simulink model "untitled"  (R2017b)
settings: Solver=FixedStepDiscrete  StartTime=0.0  StopTime=10.0  FixedStep=0.1  RelTol=1e-3  EnableMultiTasking=on
libraries: frdmk64flib x4, xpcutilitieslib x1
settings Model: ExtModeTrigDuration=5  Creator=yuy61  LastModifiedBy=chengm15
settings SolverCC: AutoInsertRateTranBlk=on
settings DataIOCC: LimitDataPoints=on
settings OptimizationCC: PassReuseOutputArgsAs=Individual arguments  MaxStackSize=64
settings DebuggingCC: ParameterTunabilityLossMsg=error  AllowSymbolicDim=off  SFUnexpectedBacktrackingDiag=warning  SFNoUnconditionalDefaultTransitionDiag=warning  SFExecutionAtInitializationDiag=none
settings HardwareCC: ProdBitPerPointer=32  ProdBitPerSizeT=32  ProdBitPerPtrDiffT=32  ProdLargestAtomicInteger=Long  ProdLargestAtomicFloat=Double  ProdWordSize=32  ProdHWDeviceType=ARM Compatible->ARM Cortex
settings SFSimCC: MATLABDynamicMemAlloc=off
settings RTWCC: SystemTargetFile=ert.tlc  HardwareBoard=NXP FRDM-K64F  TemplateMakefile=ert_default_tmf  GenerateReport=on  Toolchain=GNU Tools for ARM Embedded Processors  IncludeHyperlinkInReport=on  LaunchReport=on  GenerateTraceInfo=on  GenerateTraceReport=on  GenerateTraceReportSl=on  GenerateTraceReportSf=on  GenerateTraceReportEml=on
settings CodeAppCC: ForceParamTrailComments=on  IgnoreCustomStorageClasses=off  OperatorAnnotations=on  SimulinkDataObjDesc=on  SFDataObjDesc=on  InsertBlockDesc=on
settings ConfigComp: CovMetricSettings=dw  CovHtmlReporting=on  CovSaveCumulativeToWorkspaceVar=on  CovSaveSingleToWorkspaceVar=on  CovShowResultsExplorer=off  CovExternalEMLEnable=off  CovSFcnEnable=off

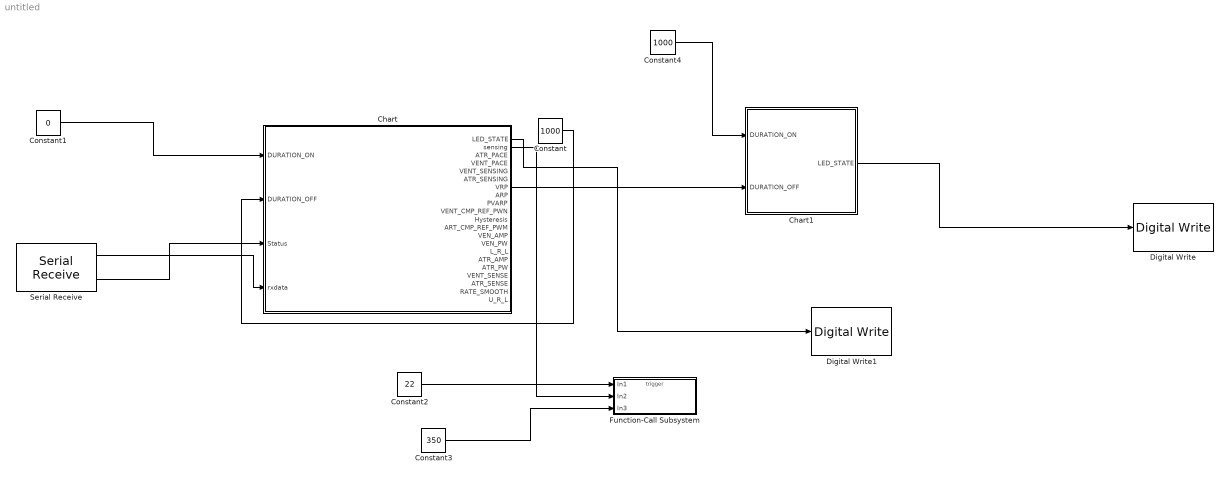
== system untitled ==
  Chart : Stateflow chart  TreatAsAtomicUnit=on
  Chart1 : Stateflow chart  TreatAsAtomicUnit=on
  Constant : Constant  Value=1000  OutDataTypeStr=int16
  Constant1 : Constant  Value=0  OutDataTypeStr=int16
  Constant2 : Constant  Value=22  OutDataTypeStr=uint8
  Constant3 : Constant  Value=350  VectorParams1D=off  OutDataTypeStr=uint16
  Constant4 : Constant  Value=1000  OutDataTypeStr=uint16
  Digital Write : frdmk64flib/Digital Write  Whichpin=RED_LED
      settings: SourceProductName=Simulink Coder Support Package for NXP FRDM-K64F Board
  Digital Write1 : frdmk64flib/Digital Write  Whichpin=GREEN_LED
      settings: SourceProductName=Simulink Coder Support Package for NXP FRDM-K64F Board
  Function-Call Subsystem : Subsystem  TreatAsAtomicUnit=on
  Serial Receive : frdmk64flib/Serial Receive  SCIModule=0  Baudrate=uint32(9600)  Parity=None  StopBits=1  HardwareFlowControl=None  ByteOrder=LittleEndian  DataType=uint8  DataLength=23  BlockingMode=off  OutputStatus=on  SampleTime=-1
      settings: SourceProductName=Simulink Coder Support Package for NXP FRDM-K64F Board
  wires:
  Constant/1 -> Chart/2(DURATION_OFF)
  Constant1/1 -> Chart/1(DURATION_ON)
  Serial Receive/2 -> Chart/3(Status)
  Serial Receive/1 -> Chart/4(rxdata)
  Chart/2(sensing) -> Function-Call Subsystem/2(In2)
  Constant2/1 -> Function-Call Subsystem/1(In1)
  Constant3/1 -> Function-Call Subsystem/3(In3)
  Chart1/1(LED_STATE) -> Digital Write/1
  Chart/7(VRP) -> Chart1/2(DURATION_OFF)
  Constant4/1 -> Chart1/1(DURATION_ON)
  Chart/1(LED_STATE) -> Digital Write1/1

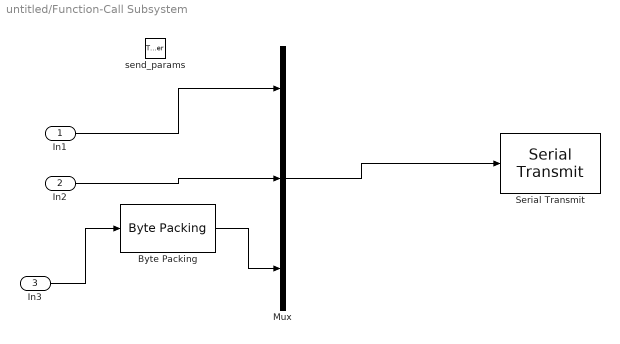
== system untitled/Function-Call Subsystem ==
  In1 : Inport  OutDataTypeStr=uint8
  In2 : Inport  Port=2  OutDataTypeStr=uint8
  In3 : Inport  Port=3  OutDataTypeStr=uint16
  send_params : TriggerPort  TriggerType=function-call  IsSimulinkFunction=on  FunctionName=send_params  VariantControl=Variant
  "Byte Packing " : xpcutilitieslib/Byte Packing   MaskPackedDataType=uint8  MaskUnpackedDataTypes={'uint16'}  MaskAlignment=1
  Mux : Mux  Inputs=3
  Serial Transmit : frdmk64flib/Serial Transmit  SCIModule=0  Baudrate=uint32(9600)  Parity=None  StopBits=1  HardwareFlowControl=None  ByteOrder=LittleEndian  BlockingMode=on  OutputStatus=off
      settings: SourceProductName=Simulink Coder Support Package for NXP FRDM-K64F Board
  wires:
  In1/1 -> Mux/1
  In2/1 -> Mux/2
  Mux/1 -> Serial Transmit/1
  In3/1 -> "Byte Packing "/1
  "Byte Packing "/1 -> Mux/3

== stateflow chart untitled/Chart1 ==
  state LED_ON
    entry:
    LED_STATE = true;
  state LED_OFF
    entry:
    LED_STATE = false;
  (default) -> LED_ON
  LED_ON -> LED_OFF : [DURATION_OFF == hex2dec('15E')]
  LED_OFF -> LED_ON : [after(DURATION_ON,msec)]
  data: DURATION_ON input uint16; DURATION_OFF input uint16; LED_STATE output boolean

== stateflow chart untitled/Chart ==
  settings: executeAtInitialization=1
  state LED_OFF
    entry:
    LED_STATE = false;
    ATR_PACE = rxdata(2)
    VENT_PACE = rxdata(3)
    ATR_SENSING = rxdata(4)
    VENT_SENSING = rxdata(5)
    VRP = typecast(rxdata(6:7), 'uint16')
    ARP = typecast(rxdata(8:9), 'uint16')
    PVARP = typecast(rxdata(10:11), 'uint16')
    Hysteresis = rxdata(12)
    VENT_CMP_REF_PWN = rxdata(13)
    ART_CMP_REF_PWM = rxdata(14)
    sensing = 1
    VEN_AMP = rxdata(15)
    VEN_PW = rxdata(16)
    U_R_L = rxdata(17)
    L_R_L = rxdata(18)
    ATR_AMP = rxdata(19)
    ATR_PW = rxdata(20)
    VENT_SENSE = rxdata(21)
    ATR_SENSE = rxdata(22)
    RATE_SMOOTH = rxdata(23)
    %sensing = 45;
    %send_params();
  state LED_ON
    entry:
    LED_STATE = true;
  state LED1
    entry:
    send_params();
  state LED
    entry:
    send_params();
  (junction 45) -> LED_OFF
  LED_ON -> (junction 45) : [Status == 0 && rxdata(1) == hex2dec('16')]
  (default) -> LED_ON
  LED_OFF -> LED_ON
  LED -> LED1 : [after(DURATION_ON,msec)]
  LED1 -> LED : [after(DURATION_ON, msec)]
  data: DURATION_ON input int16; DURATION_OFF input int16; LED_STATE output boolean; Status input uint8; rxdata input uint8; sensing output uint8; ATR_PACE output uint8; VENT_PACE output uint8; VENT_SENSING output uint8; ATR_SENSING output uint8; VRP output uint16; ARP output uint16; PVARP output uint16; VENT_CMP_REF_PWN output; Hysteresis output uint8; ART_CMP_REF_PWM output uint8; VEN_AMP output uint8; VEN_PW output uint8; L_R_L output uint8; ATR_AMP output uint8; ATR_PW output uint8; VENT_SENSE output uint8; ATR_SENSE output uint8; RATE_SMOOTH output uint8; U_R_L output uint8
